simulink model "sim01"  (R2024b)
settings: Solver=VariableStepAuto  StartTime=0.0  StopTime=20  RelTol=1e-3
values from neighbouring files (symbols this model uses):
  A = P.A    [ex_01.m]
  B = P.B    [ex_01.m]
  C = P.C    [ex_01.m]
  D = P.D    [ex_01.m]
undefined symbols (not defined in the file or in its folder): CL, K
settings Model: Creator=betot  LastModifiedBy=betot
settings OptimizationCC: ReuseModelBlockBuffer=off
settings RTWCC: GPUComputeCapability=3.5

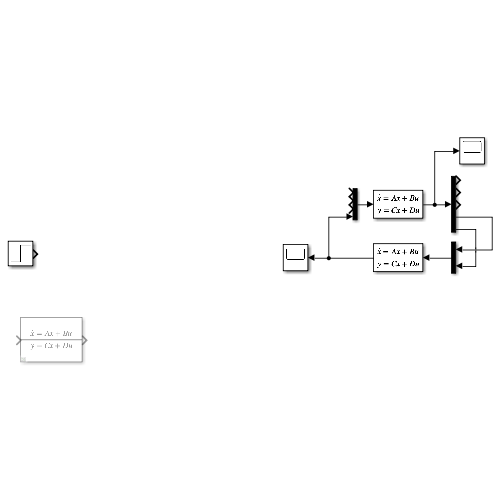
[thumbnail: Simulink's stored preview of the top-level diagram]
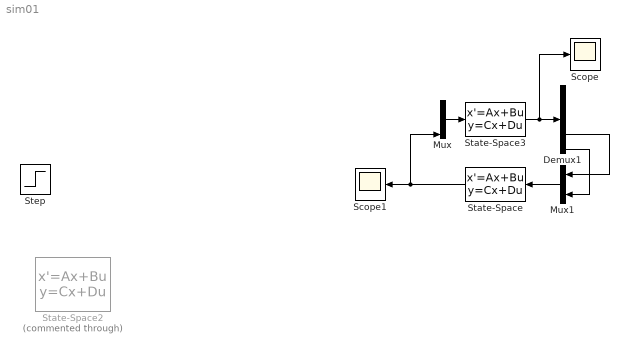
== system sim01 ==
  Demux1 : Demux  Outputs=5
  Mux : Mux
  Mux1 : Mux  Inputs=2
  Scope : Scope
  Scope1 : Scope
  State-Space : StateSpace  A=K.A  B=K.B  C=K.C  D=K.D  InitialCondition=[0; 0; 0]
  State-Space2 : StateSpace  Commented=through  A=CL.A  B=CL.B  C=CL.C  D=CL.D  InitialCondition=[0.1; 0.1; 0.1; 0.1; 0.1; 0.1]
  State-Space3 : StateSpace  A=A  B=B  C=C  D=D  InitialCondition=[5.1; 1.9; 3.1]
  Step : Step  After=0.1  SampleTime=0
  wires:
  Mux/1 -> State-Space3/1
  State-Space3/1 -> Scope/1, Demux1/1
  Mux1/1 -> State-Space/1
  Demux1/4 -> Mux1/1
  Demux1/5 -> Mux1/2
  State-Space/1 -> Scope1/1, Mux/4
